simulink model "RCAMSimulation"  (R2020b)
settings: Solver=VariableStepAuto  StartTime=0.0  StopTime=TF  RelTol=1e-3
values from neighbouring files (symbols this model uses):
  u1max = 25*pi/180    (= 0.436332312999)    [init.m]
  u1min = -25*pi/180    (= -0.436332312999)    [init.m]
  u2max = 10*pi/180    (= 0.174532925199)    [init.m]
  u2min = -25*pi/180    (= -0.436332312999)    [init.m]
  u3max = 30*pi/180    (= 0.523598775598)    [init.m]
  u3min = -30*pi/180    (= -0.523598775598)    [init.m]
  u4max = 10*pi/180    (= 0.174532925199)    [init.m]
  u4min = 0.5*pi/180*0    (= 0)    [init.m]
  u5max = 10*pi/180    (= 0.174532925199)    [init.m]
  u5min = 0.5*pi/180    (= 0.00872664625997)    [init.m]
  x0 = [85 ... (first row only)    [init.m]
undefined symbols (not defined in the file or in its folder): RCAM_model
settings Model: Creator=wilson  LastModifiedBy=wilson

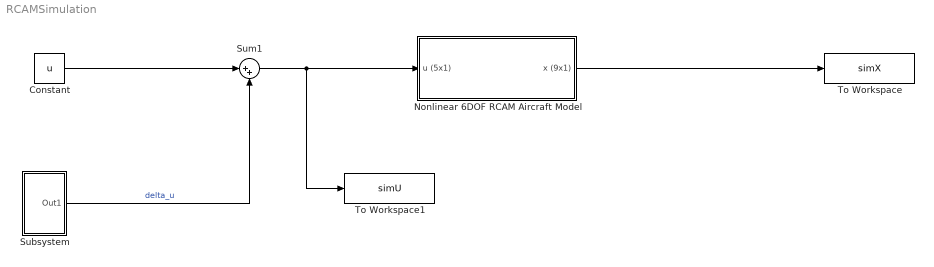
== system RCAMSimulation ==
  Constant : Constant  Value=u
  Nonlinear 6DOF RCAM Aircraft Model : Subsystem
  Subsystem : Subsystem
  Sum1 : Sum  Inputs=|++
  To Workspace : ToWorkspace  VariableName=simX  SaveFormat=Timeseries  SampleTime=-1
  To Workspace1 : ToWorkspace  VariableName=simU  SaveFormat=Timeseries  SampleTime=-1
  wires:
  Nonlinear 6DOF RCAM Aircraft Model/1(x (9x1)) -> To Workspace/1
  Constant/1 -> Sum1/1
  Subsystem/1(Out1) -> Sum1/2  "delta_u"
  Sum1/1 -> To Workspace1/1, Nonlinear 6DOF RCAM Aircraft Model/1(u (5x1))

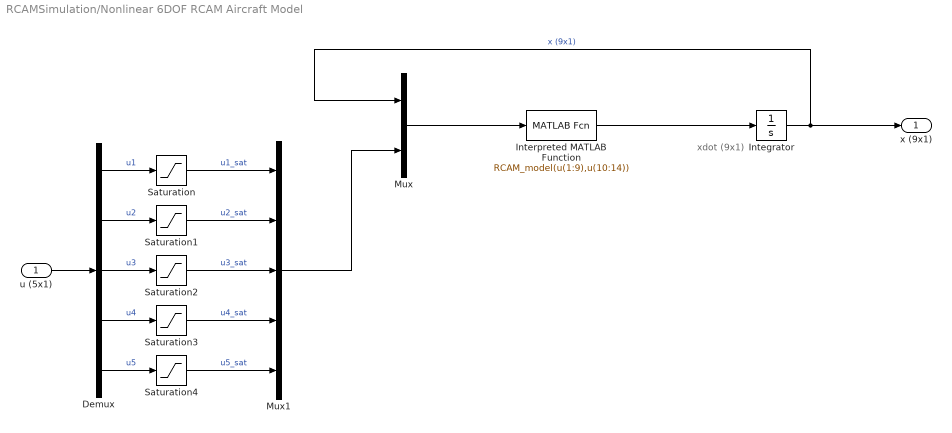
== system RCAMSimulation/Nonlinear 6DOF RCAM Aircraft Model ==
  note: xdot (9x1)
  u (5x1) : Inport
  Demux : Demux  Outputs=5
  Integrator : Integrator  InitialCondition=x0
  Interpreted MATLAB Function : MATLABFcn  MATLABFcn=RCAM_model(u(1:9),u(10:14))
  Mux : Mux  Inputs=2
  Mux1 : Mux  Inputs=5
  Saturation : Saturate  UpperLimit=u1max  LowerLimit=u1min
  Saturation1 : Saturate  UpperLimit=u2max  LowerLimit=u2min
  Saturation2 : Saturate  UpperLimit=u3max  LowerLimit=u3min
  Saturation3 : Saturate  UpperLimit=u4max  LowerLimit=u4min
  Saturation4 : Saturate  UpperLimit=u5max  LowerLimit=u5min
  x (9x1) : Outport
  wires:
  Interpreted MATLAB Function/1 -> Integrator/1
  Mux/1 -> Interpreted MATLAB Function/1
  Integrator/1 -> x (9x1)/1, Mux/1  "x (9x1)"
  u (5x1)/1 -> Demux/1
  Demux/1 -> Saturation/1  "u1"
  Saturation/1 -> Mux1/1  "u1_sat"
  Demux/2 -> Saturation1/1  "u2"
  Saturation1/1 -> Mux1/2  "u2_sat"
  Demux/3 -> Saturation2/1  "u3"
  Saturation2/1 -> Mux1/3  "u3_sat"
  Demux/4 -> Saturation3/1  "u4"
  Saturation3/1 -> Mux1/4  "u4_sat"
  Demux/5 -> Saturation4/1  "u5"
  Saturation4/1 -> Mux1/5  "u5_sat"
  Mux1/1 -> Mux/2

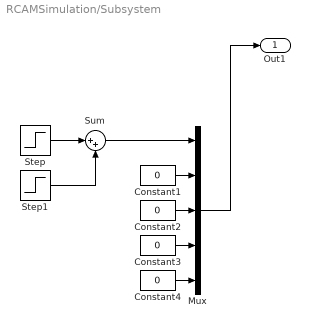
== system RCAMSimulation/Subsystem ==
  Constant{1..4} (4 alike) : Constant  Value=0
  Mux : Mux  Inputs=5
  Step : Step  Time=30  After=5*pi/180  SampleTime=0
  Step1 : Step  Time=30+2  After=-5*pi/180  SampleTime=0
  Sum : Sum  Inputs=|++
  Out1 : Outport
  wires:
  Step/1 -> Sum/1
  Constant1/1 -> Mux/2
  Step1/1 -> Sum/2
  Mux/1 -> Out1/1
  Constant4/1 -> Mux/5
  Constant2/1 -> Mux/3
  Sum/1 -> Mux/1
  Constant3/1 -> Mux/4
